simulink library "INT_EISGov_Governor"  (R2016b)
settings: Solver=VariableStepAuto  StartTime=0.0  StopTime=10.0  RelTol=1e-3
settings Model: Creator=xuxingpei  LastModifiedBy=xuxingpei

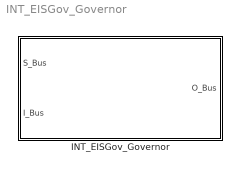
== system INT_EISGov_Governor ==
  INT_EISGov_Governor : Subsystem

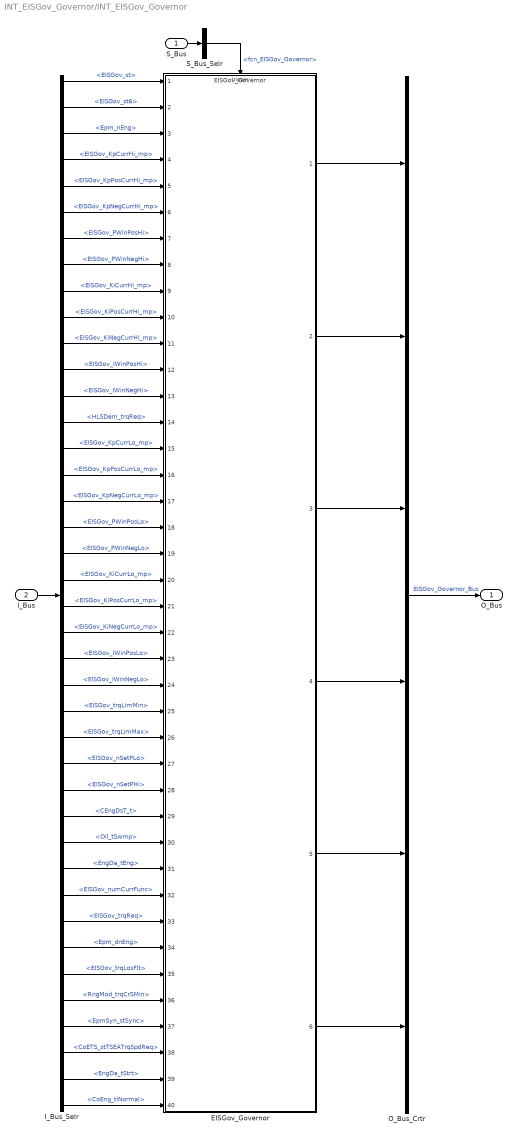
== system INT_EISGov_Governor/INT_EISGov_Governor ==
  S_Bus : Inport
  I_Bus : Inport  Port=2
  EISGov_Governor : ModelReference  ModelNameDialog=EISGov_Governor  SimulationMode=Normal  ModelReferenceVersion=1.324  TriggerPortName=function  TriggerPortTriggerType=function-call  TriggerPortStatesWhenEnabling=held
  I_Bus_Selr : BusSelector  OutputSignals=EISGov_st,EISGov_st6,Epm_nEng,EISGov_KpCurrHi_mp,EISGov_KpPosCurrHi_mp,EISGov_KpNegCurrHi_mp,EISGov_PWinPosHi,EISGov_PWinNegHi,EISGov_KiCurrHi_mp,EISGov_KiPosCurrHi_mp,EISGov_KiNegCurrHi_mp,EISGov_IWinPosHi,EISGov_IWinNegHi,HLSDem_trqReq,EISGov_KpCurrLo_mp,EISGov_KpPosCurrLo_mp,EISGov_KpNegCurrLo_mp,EISGov_PWinPosLo,EISGov_PWinNegLo,EISGov_KiCurrLo_mp,EISGov_KiPosCurrLo_mp,EISGov_KiNegCurrLo_mp,EISGov_IWinPosLo,EISGov_IWinNegLo,EISGov_trqLimMin,EISGov_trqLimMax,EISGov_nSetPLo,EISGov_nSetPHi,CEngDsT_t,Oil_tSwmp,EngDa_tEng,EISGov_numCurrFunc,EISGov_trqReq,Epm_dnEng,EISGov_trqLosFlt,RngMod_trqCrSMin,EpmSyn_stSync,CoETS_stTSEATrqSpdReq,EngDa_tStrt,CoEng_tiNormal
  O_Bus_Crtr : BusCreator  Inputs=6
  S_Bus_Selr : BusSelector  OutputSignals=fcn_EISGov_Governor
  O_Bus : Outport
  wires:
  S_Bus_Selr/1 -> EISGov_Governor/Trigger  "<fcn_EISGov_Governor>"
  S_Bus/1 -> S_Bus_Selr/1
  I_Bus/1 -> I_Bus_Selr/1
  I_Bus_Selr/1 -> EISGov_Governor/1  "<EISGov_st>"
  I_Bus_Selr/2 -> EISGov_Governor/2  "<EISGov_st6>"
  I_Bus_Selr/3 -> EISGov_Governor/3  "<Epm_nEng>"
  I_Bus_Selr/4 -> EISGov_Governor/4  "<EISGov_KpCurrHi_mp>"
  I_Bus_Selr/5 -> EISGov_Governor/5  "<EISGov_KpPosCurrHi_mp>"
  I_Bus_Selr/6 -> EISGov_Governor/6  "<EISGov_KpNegCurrHi_mp>"
  I_Bus_Selr/7 -> EISGov_Governor/7  "<EISGov_PWinPosHi>"
  I_Bus_Selr/8 -> EISGov_Governor/8  "<EISGov_PWinNegHi>"
  I_Bus_Selr/9 -> EISGov_Governor/9  "<EISGov_KiCurrHi_mp>"
  I_Bus_Selr/10 -> EISGov_Governor/10  "<EISGov_KiPosCurrHi_mp>"
  I_Bus_Selr/11 -> EISGov_Governor/11  "<EISGov_KiNegCurrHi_mp>"
  I_Bus_Selr/12 -> EISGov_Governor/12  "<EISGov_IWinPosHi>"
  I_Bus_Selr/13 -> EISGov_Governor/13  "<EISGov_IWinNegHi>"
  I_Bus_Selr/14 -> EISGov_Governor/14  "<HLSDem_trqReq>"
  I_Bus_Selr/15 -> EISGov_Governor/15  "<EISGov_KpCurrLo_mp>"
  I_Bus_Selr/16 -> EISGov_Governor/16  "<EISGov_KpPosCurrLo_mp>"
  I_Bus_Selr/17 -> EISGov_Governor/17  "<EISGov_KpNegCurrLo_mp>"
  I_Bus_Selr/18 -> EISGov_Governor/18  "<EISGov_PWinPosLo>"
  I_Bus_Selr/19 -> EISGov_Governor/19  "<EISGov_PWinNegLo>"
  I_Bus_Selr/20 -> EISGov_Governor/20  "<EISGov_KiCurrLo_mp>"
  I_Bus_Selr/21 -> EISGov_Governor/21  "<EISGov_KiPosCurrLo_mp>"
  I_Bus_Selr/22 -> EISGov_Governor/22  "<EISGov_KiNegCurrLo_mp>"
  I_Bus_Selr/23 -> EISGov_Governor/23  "<EISGov_IWinPosLo>"
  I_Bus_Selr/24 -> EISGov_Governor/24  "<EISGov_IWinNegLo>"
  I_Bus_Selr/25 -> EISGov_Governor/25  "<EISGov_trqLimMin>"
  I_Bus_Selr/26 -> EISGov_Governor/26  "<EISGov_trqLimMax>"
  I_Bus_Selr/27 -> EISGov_Governor/27  "<EISGov_nSetPLo>"
  I_Bus_Selr/28 -> EISGov_Governor/28  "<EISGov_nSetPHi>"
  I_Bus_Selr/29 -> EISGov_Governor/29  "<CEngDsT_t>"
  I_Bus_Selr/30 -> EISGov_Governor/30  "<Oil_tSwmp>"
  I_Bus_Selr/31 -> EISGov_Governor/31  "<EngDa_tEng>"
  I_Bus_Selr/32 -> EISGov_Governor/32  "<EISGov_numCurrFunc>"
  I_Bus_Selr/33 -> EISGov_Governor/33  "<EISGov_trqReq>"
  I_Bus_Selr/34 -> EISGov_Governor/34  "<Epm_dnEng>"
  I_Bus_Selr/35 -> EISGov_Governor/35  "<EISGov_trqLosFlt>"
  I_Bus_Selr/36 -> EISGov_Governor/36  "<RngMod_trqCrSMin>"
  I_Bus_Selr/37 -> EISGov_Governor/37  "<EpmSyn_stSync>"
  I_Bus_Selr/38 -> EISGov_Governor/38  "<CoETS_stTSEATrqSpdReq>"
  I_Bus_Selr/39 -> EISGov_Governor/39  "<EngDa_tStrt>"
  I_Bus_Selr/40 -> EISGov_Governor/40  "<CoEng_tiNormal>"
  O_Bus_Crtr/1 -> O_Bus/1  "EISGov_Governor_Bus"
  EISGov_Governor/1 -> O_Bus_Crtr/1
  EISGov_Governor/2 -> O_Bus_Crtr/2
  EISGov_Governor/3 -> O_Bus_Crtr/3
  EISGov_Governor/4 -> O_Bus_Crtr/4
  EISGov_Governor/5 -> O_Bus_Crtr/5
  EISGov_Governor/6 -> O_Bus_Crtr/6
